simulink model "mod_ft"  (R2021b)
settings: Solver=VariableStepAuto  StartTime=0.0  StopTime=3000  RelTol=1e-3
libraries: dsparch4 x1
settings Model: PacingRate=1000  Creator=lucas  LastModifiedBy=lucas

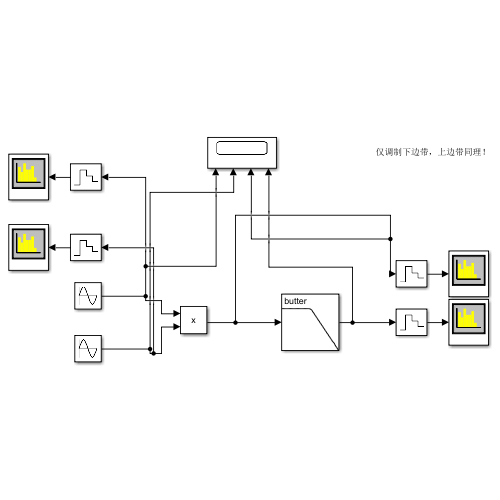
[thumbnail: Simulink's stored preview of the top-level diagram]
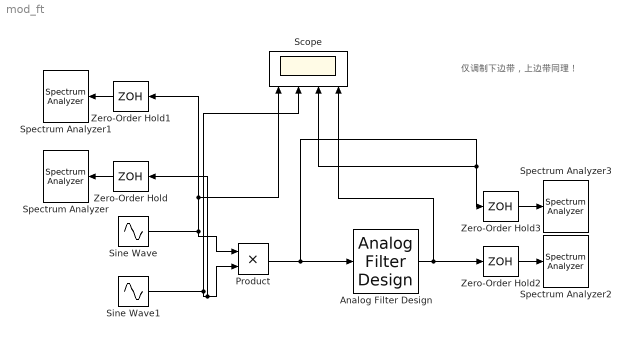
== system mod_ft ==
  note: 仅调制下边带，上边带同理！
  Analog Filter Design : dsparch4/Analog Filter Design  method=Butterworth  filttype=Lowpass  N=10  Wlo=2*pi*18  Whi=80  Rp=2  Rs=40
  Product : Product
  Scope : Scope  NumInputPorts=4
  Sine Wave : Sin  Amplitude=2  Frequency=2*pi*2  SampleTime=0
  Sine Wave1 : Sin  Amplitude=2  Frequency=2*pi*20  SampleTime=0
  Spectrum Analyzer{,1..3} (4 alike) : SpectrumAnalyzer
  Zero-Order Hold{,1..3} (4 alike) : ZeroOrderHold  SampleTime=-1
  wires:
  Sine Wave1/1 -> Zero-Order Hold/1, Product/2, Scope/2
  Sine Wave/1 -> Product/1, Zero-Order Hold1/1, Scope/1
  Analog Filter Design/1 -> Zero-Order Hold2/1, Scope/4
  Zero-Order Hold/1 -> Spectrum Analyzer/1
  Product/1 -> Zero-Order Hold3/1, Scope/3, Analog Filter Design/1
  Zero-Order Hold1/1 -> Spectrum Analyzer1/1
  Zero-Order Hold2/1 -> Spectrum Analyzer2/1
  Zero-Order Hold3/1 -> Spectrum Analyzer3/1
